simulink model "SABiR_simulator"  (Simulink 8.0)
settings: configuration reference "cset1" (kept outside this file)
values from neighbouring files (symbols this model uses):
  act_Lc_axis1 = act_Phi_axis1 \ acker(act_Phi_axis1', act_H_axis1', poles_Lpr1(1:length(act_Phi_axis1)) )'    [API_setupConstants.m]
  act_Lc_axis2 = act_Phi_axis2 \ acker(act_Phi_axis2', act_H_axis2', poles_Lpr2(1:length(act_Phi_axis2)) )'    [API_setupConstants.m]
  act_Lc_axis3 = act_Phi_axis3 \ acker(act_Phi_axis3', act_H_axis3', poles_Lpr3(1:length(act_Phi_axis3)) )'    [API_setupConstants.m]
  act_Lc_axis4 = act_Phi_axis4 \ acker(act_Phi_axis4', act_H_axis4', poles_Lpr4(1:length(act_Phi_axis4)) )'    [API_setupConstants.m]
  act_Lc_axis5 = act_Phi_axis5 \ acker(act_Phi_axis5', act_H_axis5', poles_Lpr5(1:length(act_Phi_axis5)) )'    [API_setupConstants.m]
  block1MinMax = [-20 0; -240 -180; 340 360]    [API_debugGraphs.m]    (also in API_setupConstants.m)
  block2MinMax = [-12 -7; -220 -200; 345 350]    [API_debugGraphs.m]    (also in API_setupConstants.m)
  est_Gamma_axis1 = [act_Gamma_axis1; 0]    [API_setupConstants.m]
  est_Gamma_axis2 = [act_Gamma_axis2; 0]    [API_setupConstants.m]
  est_Gamma_axis3 = [act_Gamma_axis3; 0]    [API_setupConstants.m]
  est_Gamma_axis4 = [act_Gamma_axis4; 0]    [API_setupConstants.m]
  est_Gamma_axis5 = [act_Gamma_axis5; 0]    [API_setupConstants.m]
  est_H_axis1 = [act_H_axis1, 0]    [API_setupConstants.m]
  est_H_axis2 = [act_H_axis2, 0]    [API_setupConstants.m]
  est_H_axis3 = [act_H_axis3, 0]    [API_setupConstants.m]
  est_H_axis4 = [act_H_axis4, 0]    [API_setupConstants.m]
  est_H_axis5 = [act_H_axis5, 0]    [API_setupConstants.m]
  est_Lc_axis1 = est_Phi_axis1 \ est_Lp_axis1    [API_setupConstants.m]
  est_Lc_axis2 = est_Phi_axis2 \ est_Lp_axis2    [API_setupConstants.m]
  est_Lc_axis3 = est_Phi_axis3 \ est_Lp_axis3    [API_setupConstants.m]
  est_Lc_axis4 = est_Phi_axis4 \ est_Lp_axis4    [API_setupConstants.m]
  est_Lc_axis5 = est_Phi_axis5 \ est_Lp_axis5    [API_setupConstants.m]
  est_Phi_axis1 = [act_Phi_axis1, act_Gamma_axis1; zeros(1,size(act_Phi_axis1,2)), 1]    [API_setupConstants.m]
  est_Phi_axis2 = [act_Phi_axis2, act_Gamma_axis2; zeros(1,size(act_Phi_axis2,2)), 1]    [API_setupConstants.m]
  est_Phi_axis3 = [act_Phi_axis3, act_Gamma_axis3; zeros(1,size(act_Phi_axis3,2)), 1]    [API_setupConstants.m]
  est_Phi_axis4 = [act_Phi_axis4, act_Gamma_axis4; zeros(1,size(act_Phi_axis4,2)), 1]    [API_setupConstants.m]
  est_Phi_axis5 = [act_Phi_axis5, act_Gamma_axis5; zeros(1,size(act_Phi_axis5,2)), 1]    [API_setupConstants.m]
  K_axis1 = acker(act_Phi_axis1, act_Gamma_axis1, poles_Kc1)    [API_setupConstants.m]
  K_axis2 = acker(act_Phi_axis2, act_Gamma_axis2, poles_Kc2)    [API_setupConstants.m]
  K_axis3 = acker(act_Phi_axis3, act_Gamma_axis3, poles_Kc3)    [API_setupConstants.m]
  K_axis4 = acker(act_Phi_axis4, act_Gamma_axis4, poles_Kc4)    [API_setupConstants.m]
  K_axis5 = acker(act_Phi_axis5, act_Gamma_axis5, poles_Kc5)    [API_setupConstants.m]
  Kd_dir = [0;0]    [API_setupConstants.m]
  Kd_pos = [0.0;0.0;0.0]    [API_setupConstants.m]
  Kdir = [12.5; 12.5]    [API_setupConstants.m]
  Kpos = [12.5; 12.5; 12.5]    [API_setupConstants.m]
  Nbar_axis1 = Nu_axis1 + K_axis1 * Nx_axis1    [API_setupConstants.m]
  Nbar_axis2 = Nu_axis2 + K_axis2 * Nx_axis2    [API_setupConstants.m]
  Nbar_axis3 = Nu_axis3 + K_axis3 * Nx_axis3    [API_setupConstants.m]
  Nbar_axis4 = Nu_axis4 + K_axis4 * Nx_axis4    [API_setupConstants.m]
  Nbar_axis5 = Nu_axis5 + K_axis5 * Nx_axis5    [API_setupConstants.m]
  SaturationLowerLimit = -[2;2;2;10;10;0.2]    [API_setupConstants.m]
  SaturationUpperLimit = [2;2;2;10;10;0.2]    [API_setupConstants.m]
  TorqueConstant = [TorqueConstantMotorRE25;     TorqueConstantMotorRE25;     TorqueConstantMotorRE30;     TorqueConstantMotorRE25;     TorqueConstantMotorRE25;     TorqueConstantMotorRE10]./GearRatio    [API_setupConstants.m]
  ts = 0.001    [API_relativeMove.m]    (also in API_setupConstants.m = 0.01; PosRef3D.m; PosRef3D_smooth.m; PosRefConfigSpace.m)
  ts2 = 0.0005    [API_setupConstants.m]
  tsEncoderFailure = TotalTime * encoderFailureTime    [API_simulateRobot.m]
undefined symbols (not defined in the file or in its folder): act_Gamma_axis1, act_Gamma_axis2, act_Gamma_axis3, act_Gamma_axis4, act_Gamma_axis5, act_H_axis1, act_H_axis2, act_H_axis3, act_H_axis4, act_H_axis5, act_Phi_axis1, act_Phi_axis2, act_Phi_axis3, act_Phi_axis4, act_Phi_axis5, den1, den2, den3, den4, den5, DiscIntNeverNeededParam, f_envfilt, J1_r, J2_r, J3_r, J4_r, J5_r, materialParameters1x, materialParameters2x, num1, num2, num3, num4, num5, numEncoderToFail
libraries: simulink x3
(part 1 of 3)
settings Model: Creator=M. Cenk Cavusoglu  LastModifiedBy=zhuofu
settings ConfigSet: SourceLocation=Base Workspace

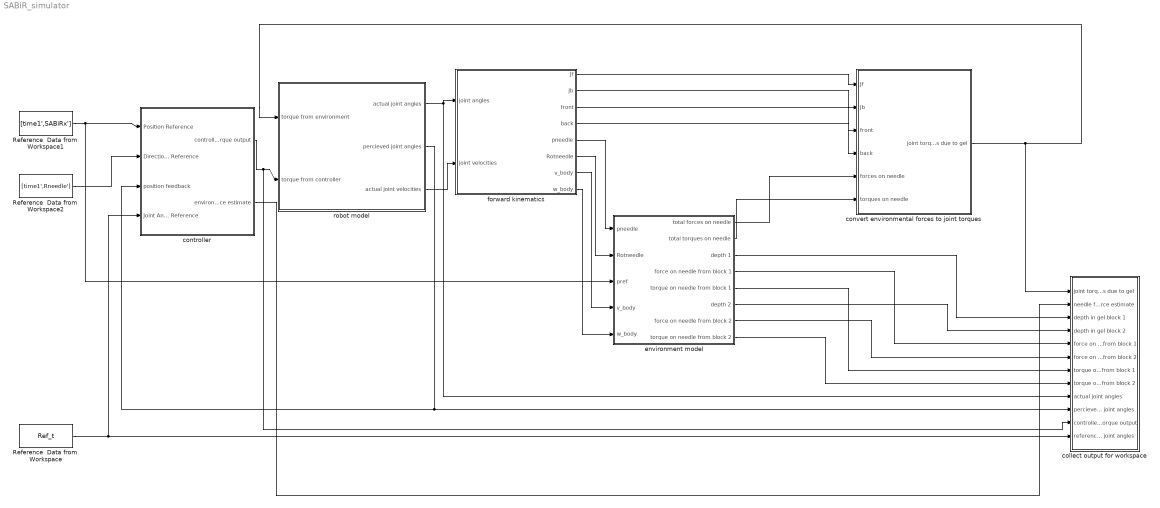
== system SABiR_simulator ==
  Reference  Data from  Workspace : FromWorkspace  VariableName=Ref_t  SampleTime=ts2  OutputAfterFinalValue=Setting to zero
  Reference  Data from  Workspace1 : FromWorkspace  VariableName=[time1',SABiRx']  SampleTime=ts2  OutputAfterFinalValue=Setting to zero
  Reference  Data from  Workspace2 : FromWorkspace  VariableName=[time1',Rneedle']  SampleTime=ts2  OutputAfterFinalValue=Setting to zero
  collect output for workspace : Subsystem
  controller : Subsystem
  convert environmental forces to joint torques : Subsystem
  environment model : Subsystem
  forward kinematics : Subsystem
  robot model : Subsystem
  wires:
  controller/1(controller torque output) -> robot model/2(torque from controller), collect output for workspace/11(controller torque output)
  robot model/2(percieved joint angles) -> collect output for workspace/10(percieved joint angles), controller/3(position feedback)
  convert environmental forces to joint torques/1(joint torques due to gel) -> robot model/1(torque from environment), collect output for workspace/1(joint torques due to gel)
  forward kinematics/1(Jf) -> convert environmental forces to joint torques/1(Jf)
  forward kinematics/2(Jb) -> convert environmental forces to joint torques/2(Jb)
  forward kinematics/5(pneedle) -> environment model/1(pneedle)
  forward kinematics/6(Rotneedle) -> environment model/2(Rotneedle)
  forward kinematics/3(front) -> convert environmental forces to joint torques/3(front)
  forward kinematics/4(back) -> convert environmental forces to joint torques/4(back)
  Reference  Data from  Workspace/1 -> collect output for workspace/12(reference joint angles), controller/4(Joint Angle Reference)
  environment model/1(total forces on needle) -> convert environmental forces to joint torques/5(forces on needle)
  environment model/2(total torques on needle) -> convert environmental forces to joint torques/6(torques on needle)
  environment model/3(depth 1) -> collect output for workspace/3(depth in gel block 1)
  environment model/4(force on needle from block 1) -> collect output for workspace/5(force on needle from block 1)
  environment model/7(force on needle from block 2) -> collect output for workspace/6(force on needle from block 2)
  environment model/5(torque on needle from block 1) -> collect output for workspace/7(torque on needle from block 1)
  environment model/8(torque on needle from block 2) -> collect output for workspace/8(torque on needle from block 2)
  environment model/6(depth 2) -> collect output for workspace/4(depth in gel block 2)
  Reference  Data from  Workspace1/1 -> controller/1(Position Reference), environment model/3(pref)
  Reference  Data from  Workspace2/1 -> controller/2(Direction Reference)
  robot model/1(actual joint angles) -> forward kinematics/1(joint angles), collect output for workspace/9(actual joint angles)
  controller/2(environment force estimate) -> collect output for workspace/2(needle force estimate)
  robot model/3(actual joint velocities) -> forward kinematics/2(joint velocities)
  forward kinematics/7(v_body) -> environment model/4(v_body)
  forward kinematics/8(w_body) -> environment model/5(w_body)

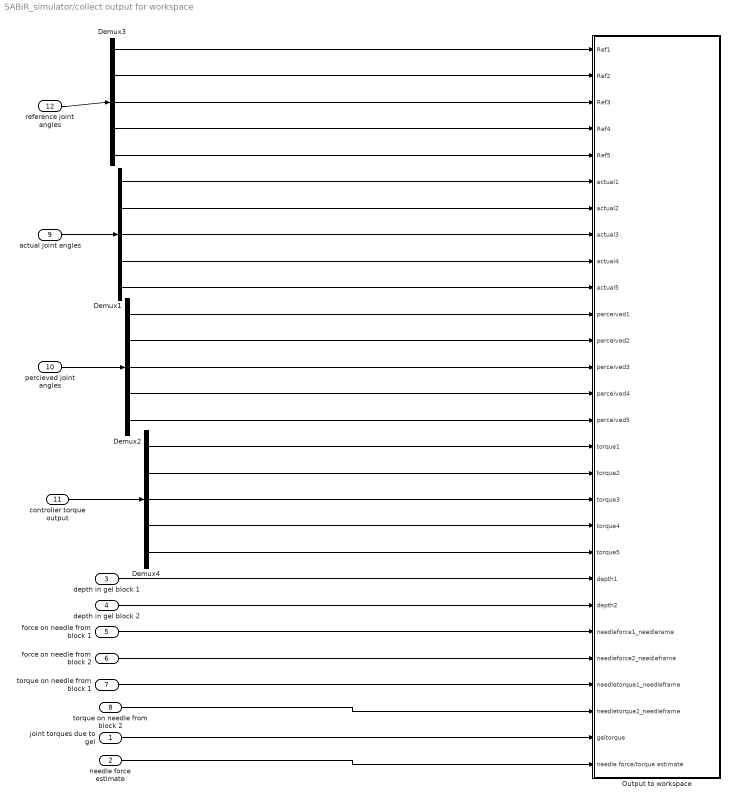
== system SABiR_simulator/collect output for workspace ==
  joint torques due to gel : Inport
  needle force estimate : Inport  Port=2
  depth in gel block 1 : Inport  Port=3
  depth in gel block 2 : Inport  Port=4
  force on needle from block 1 : Inport  Port=5
  force on needle from block 2 : Inport  Port=6
  torque on needle from block 1 : Inport  Port=7
  torque on needle from block 2 : Inport  Port=8
  actual joint angles : Inport  Port=9
  percieved joint angles : Inport  Port=10
  controller torque output : Inport  Port=11
  reference joint angles : Inport  Port=12
  Demux{1..4} (4 alike) : Demux  Outputs=5
  "Output to workspace " : Subsystem
  wires:
  reference joint angles/1 -> Demux3/1
  actual joint angles/1 -> Demux1/1
  percieved joint angles/1 -> Demux2/1
  depth in gel block 1/1 -> "Output to workspace "/21(depth1)
  depth in gel block 2/1 -> "Output to workspace "/22(depth2)
  force on needle from block 1/1 -> "Output to workspace "/23(needleforce1_needlerame)
  force on needle from block 2/1 -> "Output to workspace "/24(needleforce2_needleframe)
  torque on needle from block 1/1 -> "Output to workspace "/25(needletorque1_needleframe)
  torque on needle from block 2/1 -> "Output to workspace "/26(needletorque2_needleframe)
  joint torques due to gel/1 -> "Output to workspace "/27(geltorque)
  Demux3/1 -> "Output to workspace "/1(Ref1)
  Demux3/2 -> "Output to workspace "/2(Ref2)
  Demux3/3 -> "Output to workspace "/3(Ref3)
  Demux3/4 -> "Output to workspace "/4(Ref4)
  Demux3/5 -> "Output to workspace "/5(Ref5)
  Demux1/1 -> "Output to workspace "/6(actual1)
  Demux1/2 -> "Output to workspace "/7(actual2)
  Demux1/3 -> "Output to workspace "/8(actual3)
  Demux1/4 -> "Output to workspace "/9(actual4)
  Demux1/5 -> "Output to workspace "/10(actual5)
  Demux2/1 -> "Output to workspace "/11(perceived1)
  Demux2/2 -> "Output to workspace "/12(perceived2)
  Demux2/3 -> "Output to workspace "/13(perceived3)
  Demux2/4 -> "Output to workspace "/14(perceived4)
  Demux2/5 -> "Output to workspace "/15(perceived5)
  Demux4/1 -> "Output to workspace "/16(torque1)
  Demux4/2 -> "Output to workspace "/17(torque2)
  Demux4/3 -> "Output to workspace "/18(torque3)
  Demux4/4 -> "Output to workspace "/19(torque4)
  Demux4/5 -> "Output to workspace "/20(torque5)
  controller torque output/1 -> Demux4/1
  needle force estimate/1 -> "Output to workspace "/28(needle force/torque estimate)

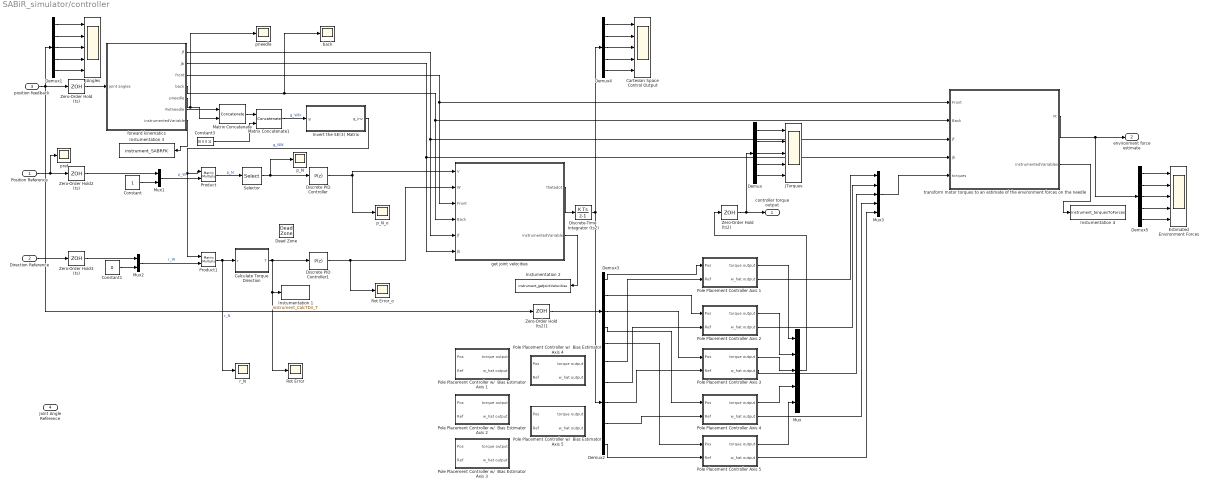
== system SABiR_simulator/controller ==
  Position Reference : Inport
  Direction Reference : Inport  Port=2
  position feedback : Inport  Port=3
  Joint Angle Reference : Inport  Port=4
  Calculate Torque Direction : MATLAB Function  TreatAsAtomicUnit=on
  Cartesian Space Control Output : Scope  NumInputPorts=5
      settings: TimeRange=5  YMin=-1~-1~-7500~-1500~-200  YMax=1~1~10000~250~1000  SaveName=ScopeData15  MaxDataPoints=50000
  Constant : Constant
  Constant1 : Constant  Value=0
  Constant3 : Constant  Value=[0 0 0 1]  VectorParams1D=off
  Dead Zone : DeadZone  LowerValue=-[0;0;0.05]  UpperValue=[0;0;0.05]  SaturateOnIntegerOverflow=on
  Demux{,1..5} (6 alike) : Demux  Outputs=5
  Discrete PID Controller : simulink/Continuous/PID Controller  Controller=P  TimeDomain=Discrete-time  SampleTime=ts  IntegratorMethod=Forward Euler  FilterMethod=Forward Euler  Form=Ideal  P=Kpos  I=0  D=Kd_pos  N=100  InitialConditionSource=internal  InitialConditionForIntegrator=0  InitialConditionForFilter=0  ExternalReset=none  LimitOutput=off  UpperSaturationLimit=inf  LowerSaturationLimit=-inf  LinearizeAsGain=off  AntiWindupMode=none  Kb=1  TrackingMode=off  Kt=1  PParamMin=[]  PParamMax=[]  IParamMin=[]  IParamMax=[]  DParamMin=[]  DParamMax=[]  NParamMin=[]  NParamMax=[]  KbParamMin=[]  KbParamMax=[]  KtParamMin=[]  KtParamMax=[]  POutMin=[]  POutMax=[]  IOutMin=[]  IOutMax=[]  DOutMin=[]  DOutMax=[]  NOutMin=[]  NOutMax=[]  KbOutMin=[]  KbOutMax=[]  KtOutMin=[]  KtOutMax=[]  IntegratorOutMin=[]  IntegratorOutMax=[]  FilterOutMin=[]  FilterOutMax=[]  SumOutMin=[]  SumOutMax=[]  SumI1OutMin=[]  SumI1OutMax=[]  SumI2OutMin=[]  SumI2OutMax=[]  SumI3OutMin=[]  SumI3OutMax=[]  SumDOutMin=[]  SumDOutMax=[]  SaturationOutMin=[]  SaturationOutMax=[]  IntegratorContinuousStateAttributes=''  IntegratorStateMustResolveToSignalObject=off  IntegratorRTWStateStorageClass=Auto  FilterContinuousStateAttributes=''  FilterStateMustResolveToSignalObject=off  FilterRTWStateStorageClass=Auto
  Discrete PID Controller1 : simulink/Continuous/PID Controller  Controller=P  TimeDomain=Discrete-time  SampleTime=ts  IntegratorMethod=Forward Euler  FilterMethod=Forward Euler  Form=Ideal  P=Kdir  I=0  D=Kd_dir  N=100  InitialConditionSource=internal  InitialConditionForIntegrator=0  InitialConditionForFilter=0  ExternalReset=none  LimitOutput=off  UpperSaturationLimit=inf  LowerSaturationLimit=-inf  LinearizeAsGain=off  AntiWindupMode=none  Kb=1  TrackingMode=off  Kt=1  PParamMin=[]  PParamMax=[]  IParamMin=[]  IParamMax=[]  DParamMin=[]  DParamMax=[]  NParamMin=[]  NParamMax=[]  KbParamMin=[]  KbParamMax=[]  KtParamMin=[]  KtParamMax=[]  POutMin=[]  POutMax=[]  IOutMin=[]  IOutMax=[]  DOutMin=[]  DOutMax=[]  NOutMin=[]  NOutMax=[]  KbOutMin=[]  KbOutMax=[]  KtOutMin=[]  KtOutMax=[]  IntegratorOutMin=[]  IntegratorOutMax=[]  FilterOutMin=[]  FilterOutMax=[]  SumOutMin=[]  SumOutMax=[]  SumI1OutMin=[]  SumI1OutMax=[]  SumI2OutMin=[]  SumI2OutMax=[]  SumI3OutMin=[]  SumI3OutMax=[]  SumDOutMin=[]  SumDOutMax=[]  SaturationOutMin=[]  SaturationOutMax=[]  IntegratorContinuousStateAttributes=''  IntegratorStateMustResolveToSignalObject=off  IntegratorRTWStateStorageClass=Auto  FilterContinuousStateAttributes=''  FilterStateMustResolveToSignalObject=off  FilterRTWStateStorageClass=Auto
  Discrete-Time Integrator (ts2) : DiscreteIntegrator  SampleTime=ts2  ICPrevOutput=DiscIntNeverNeededParam  ICPrevScaledInput=DiscIntNeverNeededParam
  Estimated Environment Forces : Scope  NumInputPorts=5
      settings: TimeRange=17.98  YMin=-5e-005~-1.75e-005~-0.0013~-0.006~-0.02  YMax=6e-005~1.25e-005~0.0001~0.004~0.0175  SaveName=ScopeData31  MaxDataPoints=50000
  Instumentation 1 : ToWorkspace  VariableName=instrument_CalcTDir_T  SampleTime=-1  SaveFormat=Structure
  Instumentation 2 : ToWorkspace  VariableName=instrument_getJointVelocities  SampleTime=-1  SaveFormat=Structure
  Instumentation 3 : ToWorkspace  VariableName=instrument_SABRFK  SampleTime=-1  SaveFormat=Structure
  Instumentation 4 : ToWorkspace  VariableName=instrument_torquesToForces  SampleTime=-1  SaveFormat=Structure
  Invert the SE(3) Matrix : MATLAB Function  TreatAsAtomicUnit=on
  JAngles : Scope  NumInputPorts=5
      settings: TimeRange=0.05  YMin=-1~-1~-3.511231084753035e-007~-1~-1  YMax=1~1~2.015504774369832e-007~1~1  SaveName=ScopeData6  MaxDataPoints=50000
  JTorques : Scope  NumInputPorts=5
      settings: TimeRange=18  YMin=-0.00025~-0.0003~-0.0003~-0.0007~-0.00075  YMax=0.0002~0.0003~0.00015~0.0004~0.001  SaveName=ScopeData3  MaxDataPoints=50000
  Matrix Concatenate : Concatenate  Mode=Multidimensional array  ConcatenateDimension=2
  Matrix Concatenate1 : Concatenate  Mode=Multidimensional array
  Mux : Mux  Inputs=5
  Mux1 : Mux  Inputs=[3 1]
  Mux2 : Mux  Inputs=[3 1]
  Mux3 : Mux  Inputs=5
  Pole Placement Controller Axis 1 : Subsystem
  Pole Placement Controller Axis 2 : Subsystem
  Pole Placement Controller Axis 3 : Subsystem
  Pole Placement Controller Axis 4 : Subsystem
  Pole Placement Controller Axis 5 : Subsystem
  Pole Placement Controller w/  Bias Estimator Axis 1 : Subsystem
  Pole Placement Controller w/  Bias Estimator Axis 2 : Subsystem
  Pole Placement Controller w/  Bias Estimator Axis 3 : Subsystem
  Pole Placement Controller w/  Bias Estimator Axis 4 : Subsystem
  Pole Placement Controller w/  Bias Estimator Axis 5 : Subsystem
  Product : Product  Multiplication=Matrix(*)  RndMeth=Zero
  Product1 : Product  Multiplication=Matrix(*)  RndMeth=Zero
  Rot Error : Scope
      settings: TimeRange=12  YMin=-0.15  YMax=0.55  SaveName=ScopeData2  MaxDataPoints=50000
  Rot Error_o : Scope
      settings: TimeRange=5  YMin=-150  YMax=100  SaveName=ScopeData17  MaxDataPoints=50000
  Selector : Selector  InputPortWidth=4  IndexOptions=Index vector (dialog)  Indices=[1 2 3]  OutputSizes=1
  Zero-Order Hold (ts) : ZeroOrderHold  SampleTime=ts
  Zero-Order Hold (ts2) : ZeroOrderHold  SampleTime=ts2
  Zero-Order Hold (ts2)1 : ZeroOrderHold  SampleTime=ts2
  Zero-Order Hold2 (ts) : ZeroOrderHold  SampleTime=ts
  Zero-Order Hold3 (ts) : ZeroOrderHold  SampleTime=ts
  back : Scope
      settings: TimeRange=5  YMin=-150  YMax=100  SaveName=ScopeData5  MaxDataPoints=50000
  forward kinematics : Subsystem
  get joint velocities : MATLAB Function  TreatAsAtomicUnit=on
  p_N : Scope
      settings: TimeRange=17.98  YMin=-0.55  YMax=0.55  MaxDataPoints=50000
  p_N_o : Scope
      settings: TimeRange=5  YMin=-150  YMax=100  SaveName=ScopeData16  MaxDataPoints=50000
  pneedle : Scope
      settings: TimeRange=17.98  YMin=-225  YMax=350  SaveName=ScopeData4  MaxDataPoints=50000
  pref : Scope
      settings: TimeRange=17.98  YMin=-225  YMax=350  SaveName=ScopeData21  MaxDataPoints=50000
  r_N : Scope
      settings: TimeRange=5  YMin=-150  YMax=100  MaxDataPoints=50000
  transform motor torques to an estimate of the environment forces on the needle : MATLAB Function  TreatAsAtomicUnit=on
  controller torque output : Outport
  environment force estimate : Outport  Port=2
  wires:
  Position Reference/1 -> Zero-Order Hold2 (ts)/1, pref/1
  position feedback/1 -> Zero-Order Hold (ts)/1, Demux1/1, Zero-Order Hold (ts2)1/1
  Direction Reference/1 -> Zero-Order Hold3 (ts)/1
  Matrix Concatenate1/1 -> Invert the SE(3) Matrix/1(g)  "g_WN"
  Zero-Order Hold2 (ts)/1 -> Mux1/1
  Constant/1 -> Mux1/2
  Invert the SE(3) Matrix/1(g_inv) -> Product/1, Product1/1  "g_NW"
  Mux1/1 -> Product/2  "p_W"
  Product/1 -> Selector/1  "p_N"
  Selector/1 -> p_N/1, Discrete PID Controller/1
  Constant1/1 -> Mux2/2
  Zero-Order Hold3 (ts)/1 -> Mux2/1
  Mux2/1 -> Product1/2  "r_W"
  Product1/1 -> Calculate Torque Direction/1(r), r_N/1  "r_N"
  Calculate Torque Direction/1(T) -> Discrete PID Controller1/1, Rot Error/1, Instumentation 1/1
  Discrete PID Controller1/1 -> Rot Error_o/1, get joint velocities/2(W)
  forward kinematics/3(front) -> get joint velocities/3(Front), transform motor torques to an estimate of the environment forces on the needle/1(Front)
  forward kinematics/4(back) -> back/1, get joint velocities/4(Back), transform motor torques to an estimate of the environment forces on the needle/2(Back)
  forward kinematics/1(Jf) -> get joint velocities/5(Jf), transform motor torques to an estimate of the environment forces on the needle/3(Jf)
  forward kinematics/2(Jb) -> get joint velocities/6(Jb), transform motor torques to an estimate of the environment forces on the needle/4(Jb)
  forward kinematics/6(Rotneedle) -> Matrix Concatenate/1
  forward kinematics/5(pneedle) -> pneedle/1, Matrix Concatenate/2
  Matrix Concatenate/1 -> Matrix Concatenate1/1
  Constant3/1 -> Matrix Concatenate1/2
  Demux/5 -> JTorques/5
  Demux/4 -> JTorques/4
  Demux/3 -> JTorques/3
  Demux/2 -> JTorques/2
  Demux/1 -> JTorques/1
  Demux1/5 -> JAngles/5
  Demux1/4 -> JAngles/4
  Demux1/3 -> JAngles/3
  Demux1/2 -> JAngles/2
  Demux1/1 -> JAngles/1
  Discrete PID Controller/1 -> p_N_o/1, get joint velocities/1(V)
  Pole Placement Controller Axis 4/1(torque output) -> Mux/4
  Pole Placement Controller Axis 5/1(torque output) -> Mux/5
  Pole Placement Controller Axis 3/1(torque output) -> Mux/3
  Pole Placement Controller Axis 2/1(torque output) -> Mux/2
  Pole Placement Controller Axis 1/1(torque output) -> Mux/1
  Demux2/5 -> Pole Placement Controller Axis 5/2(Ref)
  Demux2/4 -> Pole Placement Controller Axis 4/2(Ref)
  Demux2/3 -> Pole Placement Controller Axis 3/2(Ref)
  Demux2/2 -> Pole Placement Controller Axis 2/2(Ref)
  Demux2/1 -> Pole Placement Controller Axis 1/2(Ref)
  Demux3/1 -> Pole Placement Controller Axis 1/1(Pos)
  Demux3/2 -> Pole Placement Controller Axis 2/1(Pos)
  Demux3/3 -> Pole Placement Controller Axis 3/1(Pos)
  Demux3/4 -> Pole Placement Controller Axis 4/1(Pos)
  Demux3/5 -> Pole Placement Controller Axis 5/1(Pos)
  Demux4/5 -> Cartesian Space Control Output/5
  Demux4/4 -> Cartesian Space Control Output/4
  Demux4/3 -> Cartesian Space Control Output/3
  Demux4/2 -> Cartesian Space Control Output/2
  Demux4/1 -> Cartesian Space Control Output/1
  Zero-Order Hold (ts2)/1 -> controller torque output/1, Demux/1
  Mux/1 -> Zero-Order Hold (ts2)/1
  get joint velocities/1(thetadot) -> Discrete-Time Integrator (ts2)/1
  Discrete-Time Integrator (ts2)/1 -> Demux4/1, Demux2/1
  Zero-Order Hold (ts)/1 -> forward kinematics/1(joint angles)
  Zero-Order Hold (ts2)1/1 -> Demux3/1
  transform motor torques to an estimate of the environment forces on the needle/1(Ft) -> environment force estimate/1, Demux5/1
  Mux3/1 -> transform motor torques to an estimate of the environment forces on the needle/5(torques)
  Pole Placement Controller Axis 5/2(w_hat output) -> Mux3/5
  Pole Placement Controller Axis 4/2(w_hat output) -> Mux3/4
  Pole Placement Controller Axis 2/2(w_hat output) -> Mux3/2
  Pole Placement Controller Axis 1/2(w_hat output) -> Mux3/1
  Pole Placement Controller Axis 3/2(w_hat output) -> Mux3/3
  Demux5/5 -> Estimated Environment Forces/5
  Demux5/4 -> Estimated Environment Forces/4
  Demux5/3 -> Estimated Environment Forces/3
  Demux5/2 -> Estimated Environment Forces/2
  Demux5/1 -> Estimated Environment Forces/1
  get joint velocities/2(instrumentedVariable) -> Instumentation 2/1
  transform motor torques to an estimate of the environment forces on the needle/2(instrumentedVariables) -> Instumentation 4/1
  forward kinematics/7(instrumentedVariable) -> Instumentation 3/1

== system SABiR_simulator/convert environmental forces to joint torques ==
  Jf : Inport
  Jb : Inport  Port=2
  front : Inport  Port=3
  back : Inport  Port=4
  forces on needle : Inport  Port=5
  torques on needle : Inport  Port=6
  Demux1 : Demux  Outputs=3
  Demux2 : Demux  Outputs=3
  Env Forces on Needle : Scope  NumInputPorts=3
      settings: TimeRange=17.98  YMin=-7.5e-007~-7e-007~-0.0013  YMax=2e-006~3e-007~0.0001  SaveName=ScopeData32  MaxDataPoints=50000
  Env Torques on Needle : Scope  NumInputPorts=3
      settings: TimeRange=17.98  YMin=-2.75e-008~-1.2e-007~-1e-008  YMax=1e-008~1e-008~5e-009  SaveName=ScopeData33  MaxDataPoints=50000
  Motor Torques Due to Environment Forces : Scope
      settings: TimeRange=17.98  YMin=-1  YMax=1  SaveName=ScopeData22  MaxDataPoints=50000
  get joint torques : MATLAB Function  TreatAsAtomicUnit=on
  joint torques due to gel : Outport
  wires:
  forces on needle/1 -> get joint torques/1(F), Demux2/1
  torques on needle/1 -> get joint torques/2(T), Demux1/1
  front/1 -> get joint torques/3(Front)
  back/1 -> get joint torques/4(Back)
  Jf/1 -> get joint torques/5(Jf)
  Jb/1 -> get joint torques/6(Jb)
  get joint torques/1(torques) -> joint torques due to gel/1, Motor Torques Due to Environment Forces/1
  Demux1/3 -> Env Torques on Needle/3
  Demux1/2 -> Env Torques on Needle/2
  Demux1/1 -> Env Torques on Needle/1
  Demux2/3 -> Env Forces on Needle/3
  Demux2/2 -> Env Forces on Needle/2
  Demux2/1 -> Env Forces on Needle/1

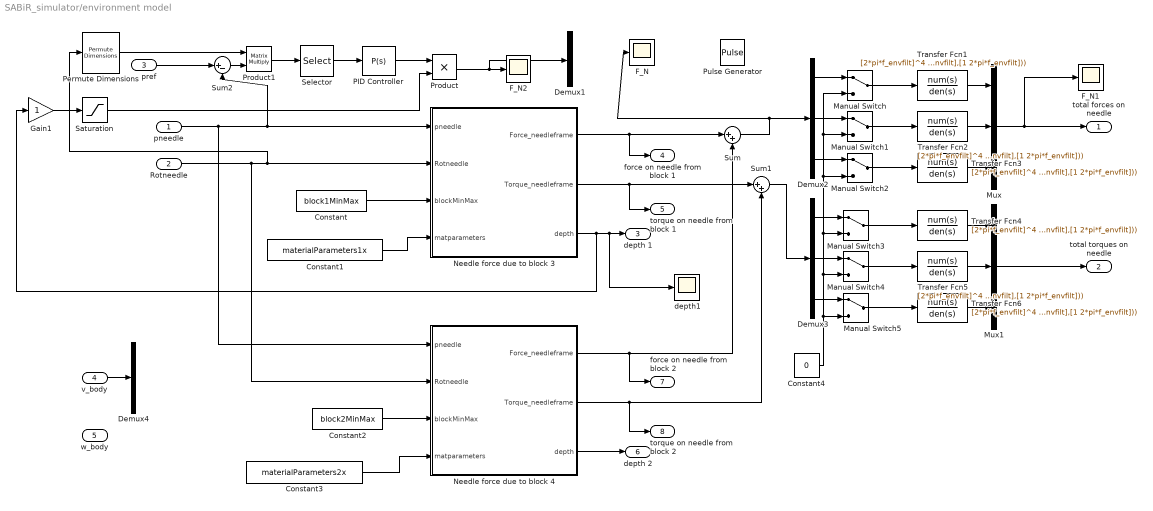
== system SABiR_simulator/environment model ==
  pneedle : Inport
  Rotneedle : Inport  Port=2
  pref : Inport  Port=3
  v_body : Inport  Port=4
  w_body : Inport  Port=5
  Constant : Constant  Value=block1MinMax  VectorParams1D=off
  Constant1 : Constant  Value=materialParameters1x  VectorParams1D=off
  Constant2 : Constant  Value=block2MinMax  VectorParams1D=off
  Constant3 : Constant  Value=materialParameters2x  VectorParams1D=off
  Constant4 : Constant  Value=0
  Demux1 : Demux  Outputs=2
  Demux2 : Demux  Outputs=3
  Demux3 : Demux  Outputs=3
  Demux4 : Demux  Outputs=3
  F_N : Scope
      settings: TimeRange=5  YMin=-0.175  YMax=0.1  SaveName=ScopeData23  MaxDataPoints=50000
  F_N1 : Scope
      settings: TimeRange=17.98  YMin=-1  YMax=1  SaveName=ScopeData24  MaxDataPoints=50000
  F_N2 : Scope
      settings: TimeRange=5  YMin=-1.75e-005  YMax=1.75e-005  SaveName=ScopeData26  MaxDataPoints=50000
  Gain1 : Gain
  Manual Switch{,1..5} (6 alike) : ManualSwitch
  Mux : Mux  Inputs=3
  Mux1 : Mux  Inputs=3
  Needle force due to block 3 : Subsystem
  Needle force due to block 4 : Subsystem
  PID Controller : simulink/Continuous/PID Controller  Controller=P  TimeDomain=Continuous-time  SampleTime=1  IntegratorMethod=Forward Euler  FilterMethod=Forward Euler  Form=Ideal  P=0.0087/25  I=0  D=0  N=100  InitialConditionSource=internal  InitialConditionForIntegrator=0  InitialConditionForFilter=0  ExternalReset=none  LimitOutput=off  UpperSaturationLimit=inf  LowerSaturationLimit=-inf  LinearizeAsGain=off  AntiWindupMode=none  Kb=1  TrackingMode=off  Kt=1  PParamMin=[]  PParamMax=[]  IParamMin=[]  IParamMax=[]  DParamMin=[]  DParamMax=[]  NParamMin=[]  NParamMax=[]  KbParamMin=[]  KbParamMax=[]  KtParamMin=[]  KtParamMax=[]  POutMin=[]  POutMax=[]  IOutMin=[]  IOutMax=[]  DOutMin=[]  DOutMax=[]  NOutMin=[]  NOutMax=[]  KbOutMin=[]  KbOutMax=[]  KtOutMin=[]  KtOutMax=[]  IntegratorOutMin=[]  IntegratorOutMax=[]  FilterOutMin=[]  FilterOutMax=[]  SumOutMin=[]  SumOutMax=[]  SumI1OutMin=[]  SumI1OutMax=[]  SumI2OutMin=[]  SumI2OutMax=[]  SumI3OutMin=[]  SumI3OutMax=[]  SumDOutMin=[]  SumDOutMax=[]  SaturationOutMin=[]  SaturationOutMax=[]  IntegratorContinuousStateAttributes=''  IntegratorStateMustResolveToSignalObject=off  IntegratorRTWStateStorageClass=Auto  FilterContinuousStateAttributes=''  FilterStateMustResolveToSignalObject=off  FilterRTWStateStorageClass=Auto
  Permute Dimensions : PermuteDimensions
  Product : Product  RndMeth=Zero
  Product1 : Product  Multiplication=Matrix(*)  RndMeth=Zero
  Pulse Generator : DiscretePulseGenerator  PulseType=Time based  Amplitude=1e-5  Period=1  PulseWidth=5
  Saturation : Saturate  UpperLimit=20  LowerLimit=0
  Selector : Selector  InputPortWidth=3  IndexOptions=Index vector (dialog)  Indices=[1 2]  OutputSizes=1
  Sum : Sum  Inputs=|++
  Sum1 : Sum  Inputs=|++
  Sum2 : Sum  Inputs=|+-
  Transfer Fcn{1..6} (6 alike) : TransferFcn  Numerator=[2*pi*f_envfilt]^4  Denominator=conv(conv([1 2*pi*f_envfilt],[1 2*pi*f_envfilt]),conv([1 2*pi*f_envfilt],[1 2*pi*f_envfilt]))
  depth1 : Scope
      settings: TimeRange=5  YMin=-0.175  YMax=0.1  SaveName=ScopeData25  MaxDataPoints=50000
  total forces on needle : Outport
  total torques on needle : Outport  Port=2
  depth 1 : Outport  Port=3
  force on needle from block 1 : Outport  Port=4
  torque on needle from block 1 : Outport  Port=5
  depth 2 : Outport  Port=6
  force on needle from block 2 : Outport  Port=7
  torque on needle from block 2 : Outport  Port=8
  wires:
  pneedle/1 -> Sum2/2, Needle force due to block 3/1(pneedle), Needle force due to block 4/1(pneedle)
  Rotneedle/1 -> Permute Dimensions/1, Needle force due to block 3/2(Rotneedle), Needle force due to block 4/2(Rotneedle)
  Needle force due to block 3/3(depth) -> Gain1/1, depth 1/1, depth1/1
  Needle force due to block 3/1(Force_needleframe) -> Sum/1, force on needle from block 1/1
  Needle force due to block 3/2(Torque_needleframe) -> Sum1/1, torque on needle from block 1/1
  Needle force due to block 4/3(depth) -> depth 2/1
  Needle force due to block 4/1(Force_needleframe) -> force on needle from block 2/1, Sum/2
  Needle force due to block 4/2(Torque_needleframe) -> torque on needle from block 2/1, Sum1/2
  Constant/1 -> Needle force due to block 3/3(blockMinMax)
  Constant2/1 -> Needle force due to block 4/3(blockMinMax)
  Constant3/1 -> Needle force due to block 4/4(matparameters)
  Mux/1 -> F_N1/1, total forces on needle/1
  Mux1/1 -> total torques on needle/1
  Manual Switch/1 -> Transfer Fcn1/1
  Manual Switch1/1 -> Transfer Fcn2/1
  Manual Switch3/1 -> Transfer Fcn4/1
  Manual Switch4/1 -> Transfer Fcn5/1
  Manual Switch5/1 -> Transfer Fcn6/1
  Sum1/1 -> Demux3/1
  Sum/1 -> F_N/1, Demux2/1
  Demux2/3 -> Manual Switch2/1
  Demux3/1 -> Manual Switch3/1
  Demux3/2 -> Manual Switch4/1
  Demux3/3 -> Manual Switch5/1
  Constant4/1 -> Manual Switch5/2, Manual Switch4/2, Manual Switch3/2, Manual Switch2/2, Manual Switch1/2, Manual Switch/2
  Saturation/1 -> Product/2
  PID Controller/1 -> Product/1
  Product/1 -> F_N2/1, Demux1/1
  Gain1/1 -> Saturation/1
  Selector/1 -> PID Controller/1
  Product1/1 -> Selector/1
  Sum2/1 -> Product1/2
  Permute Dimensions/1 -> Product1/1
  pref/1 -> Sum2/1
  Constant1/1 -> Needle force due to block 3/4(matparameters)
  Demux2/2 -> Manual Switch1/1
  Demux2/1 -> Manual Switch/1
  Manual Switch2/1 -> Transfer Fcn3/1
  v_body/1 -> Demux4/1
  Transfer Fcn1/1 -> Mux/1
  Transfer Fcn2/1 -> Mux/2
  Transfer Fcn3/1 -> Mux/3
  Transfer Fcn4/1 -> Mux1/1
  Transfer Fcn5/1 -> Mux1/2
  Transfer Fcn6/1 -> Mux1/3

== system SABiR_simulator/forward kinematics ==
  joint angles : Inport
  joint velocities : Inport  Port=2
  Bus Selector : BusSelector  OutputSignals=signal1,signal2,signal3,signal4,signal5
  Demux4 : Demux  Outputs=6
  Needle Body Velociy : Scope  NumInputPorts=5
      settings: TimeRange=17.98  YMin=-45~-10~-125~-0.07~-0.3  YMax=40~10~100~0.06~0.3  SaveName=ScopeData28  MaxDataPoints=50000
  forward kinematics1 : MATLAB Function  TreatAsAtomicUnit=on
  get joint velocities : MATLAB Function  TreatAsAtomicUnit=on
  Jf : Outport
  Jb : Outport  Port=2
  front : Outport  Port=3
  back : Outport  Port=4
  pneedle : Outport  Port=5
  Rotneedle : Outport  Port=6
  v_body : Outport  Port=7
  w_body : Outport  Port=8
  wires:
  forward kinematics1/1(NeedleTip) -> pneedle/1
  forward kinematics1/3(Front) -> front/1, get joint velocities/2(Front)
  forward kinematics1/4(Back) -> back/1, get joint velocities/3(Back)
  forward kinematics1/5(Jf) -> Jf/1, get joint velocities/4(Jf)
  forward kinematics1/6(Jb) -> Jb/1, get joint velocities/5(Jb)
  forward kinematics1/2(NeedleRot) -> Rotneedle/1
  joint angles/1 -> Bus Selector/1
  Bus Selector/1 -> forward kinematics1/1(t1)  "<signal1>"
  Bus Selector/2 -> forward kinematics1/2(t2)  "<signal2>"
  Bus Selector/3 -> forward kinematics1/3(t3)  "<signal3>"
  Bus Selector/4 -> forward kinematics1/4(t4)  "<signal4>"
  Bus Selector/5 -> forward kinematics1/5(t5)  "<signal5>"
  joint velocities/1 -> get joint velocities/1(thetadot)
  get joint velocities/2(wb) -> w_body/1
  get joint velocities/1(vb) -> v_body/1
  Demux4/5 -> Needle Body Velociy/5
  Demux4/4 -> Needle Body Velociy/4
  Demux4/3 -> Needle Body Velociy/3
  Demux4/2 -> Needle Body Velociy/2
  Demux4/1 -> Needle Body Velociy/1
  get joint velocities/3(bodyVel) -> Demux4/1

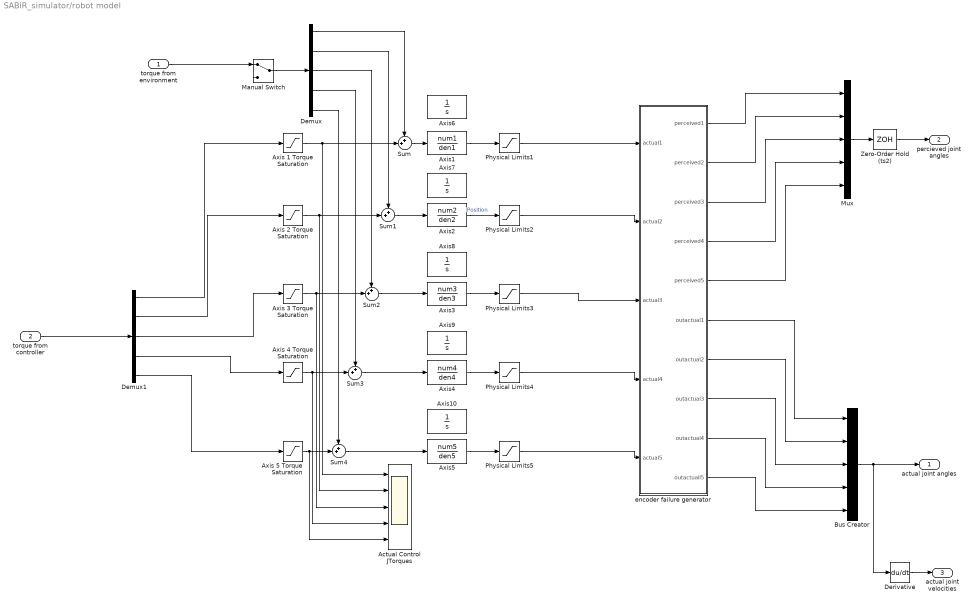
== system SABiR_simulator/robot model ==
  torque from environment : Inport
  torque from controller : Inport  Port=2
  Actual Control JTorques : Scope  NumInputPorts=5
      settings: TimeRange=5  YMin=-0.0001~-2e-005~-1e-005~-0.0003~-7.5e-005  YMax=0.000225~0.00014~0.00011~0.0008~0.000275  SaveName=ScopeData20  MaxDataPoints=50000
  Axis 1 Torque Saturation : Saturate  UpperLimit=SaturationUpperLimit(1)./(1./TorqueConstant(1))  LowerLimit=SaturationLowerLimit(1)./(1./TorqueConstant(1))
  Axis 2 Torque Saturation : Saturate  UpperLimit=SaturationUpperLimit(2)./(1./TorqueConstant(2))  LowerLimit=SaturationLowerLimit(2)./(1./TorqueConstant(2))
  Axis 3 Torque Saturation : Saturate  UpperLimit=SaturationUpperLimit(3)./(1./TorqueConstant(3))  LowerLimit=SaturationLowerLimit(3)./(1./TorqueConstant(3))
  Axis 4 Torque Saturation : Saturate  UpperLimit=SaturationUpperLimit(4)./(1./TorqueConstant(4))  LowerLimit=SaturationLowerLimit(4)./(1./TorqueConstant(4))
  Axis 5 Torque Saturation : Saturate  UpperLimit=SaturationUpperLimit(5)./(1./TorqueConstant(5))  LowerLimit=SaturationLowerLimit(5)./(1./TorqueConstant(5))
  Axis1 : TransferFcn  Numerator=num1  Denominator=den1
  Axis10 : TransferFcn  Denominator=[1 0]
  Axis2 : TransferFcn  Numerator=num2  Denominator=den2
  Axis3 : TransferFcn  Numerator=num3  Denominator=den3  ContinuousStateAttributes='tf3'
  Axis4 : TransferFcn  Numerator=num4  Denominator=den4
  Axis5 : TransferFcn  Numerator=num5  Denominator=den5
  Axis{6..9} (4 alike) : TransferFcn  Numerator=1  Denominator=[1 0]
  Bus Creator : BusCreator  Inputs=5
  Demux : Demux  Outputs=5
  Demux1 : Demux  Outputs=5
  Derivative : Derivative
  Manual Switch : ManualSwitch
  Mux : Mux  Inputs=5
  Physical Limits1 : Saturate  UpperLimit=0.7854  LowerLimit=-0.5060
  Physical Limits2 : Saturate  UpperLimit=0.4841  LowerLimit=-0.7854
  Physical Limits3 : Saturate  UpperLimit=0.2961*100  LowerLimit=-0.2618*100
  Physical Limits4 : Saturate  UpperLimit=0.7854  LowerLimit=-0.4531
  Physical Limits5 : Saturate  UpperLimit=0.4396  LowerLimit=-0.7854
  Sum{,1..4} (5 alike) : Sum  Inputs=++|
  Zero-Order Hold (ts2) : ZeroOrderHold  SampleTime=ts2
  encoder failure generator : Subsystem
  actual joint angles : Outport
  percieved joint angles : Outport  Port=2
  actual joint velocities : Outport  Port=3
  wires:
  Axis 3 Torque Saturation/1 -> Sum2/2, Actual Control JTorques/3
  Physical Limits1/1 -> encoder failure generator/1(actual1)
  Physical Limits2/1 -> encoder failure generator/2(actual2)
  Physical Limits4/1 -> encoder failure generator/4(actual4)
  Physical Limits5/1 -> encoder failure generator/5(actual5)
  torque from controller/1 -> Demux1/1
  Demux1/3 -> Axis 3 Torque Saturation/1
  Demux/1 -> Sum/1
  Demux/2 -> Sum1/1
  Demux/3 -> Sum2/1
  Demux/4 -> Sum3/1
  Demux/5 -> Sum4/1
  Axis 1 Torque Saturation/1 -> Sum/2, Actual Control JTorques/1
  Axis 2 Torque Saturation/1 -> Sum1/2, Actual Control JTorques/2
  Axis 4 Torque Saturation/1 -> Sum3/2, Actual Control JTorques/4
  Axis 5 Torque Saturation/1 -> Sum4/2, Actual Control JTorques/5
  Mux/1 -> Zero-Order Hold (ts2)/1
  encoder failure generator/1(perceived1) -> Mux/1
  encoder failure generator/2(perceived2) -> Mux/2
  encoder failure generator/3(perceived3) -> Mux/3
  encoder failure generator/4(perceived4) -> Mux/4
  encoder failure generator/5(perceived5) -> Mux/5
  Physical Limits3/1 -> encoder failure generator/3(actual3)
  Zero-Order Hold (ts2)/1 -> percieved joint angles/1
  torque from environment/1 -> Manual Switch/1
  Manual Switch/1 -> Demux/1
  Demux1/5 -> Axis 5 Torque Saturation/1
  Demux1/4 -> Axis 4 Torque Saturation/1
  Demux1/2 -> Axis 2 Torque Saturation/1
  Demux1/1 -> Axis 1 Torque Saturation/1
  Sum/1 -> Axis1/1
  Axis1/1 -> Physical Limits1/1
  Sum1/1 -> Axis2/1
  Axis2/1 -> Physical Limits2/1  "Position"
  Sum2/1 -> Axis3/1
  Axis3/1 -> Physical Limits3/1
  Sum3/1 -> Axis4/1
  Axis4/1 -> Physical Limits4/1
  Sum4/1 -> Axis5/1
  Axis5/1 -> Physical Limits5/1
  encoder failure generator/6(outactual1) -> Bus Creator/1
  encoder failure generator/7(outactual2) -> Bus Creator/2
  encoder failure generator/8(outactual3) -> Bus Creator/3
  encoder failure generator/9(outactual4) -> Bus Creator/4
  encoder failure generator/10(outactuall5) -> Bus Creator/5
  Bus Creator/1 -> actual joint angles/1, Derivative/1
  Derivative/1 -> actual joint velocities/1

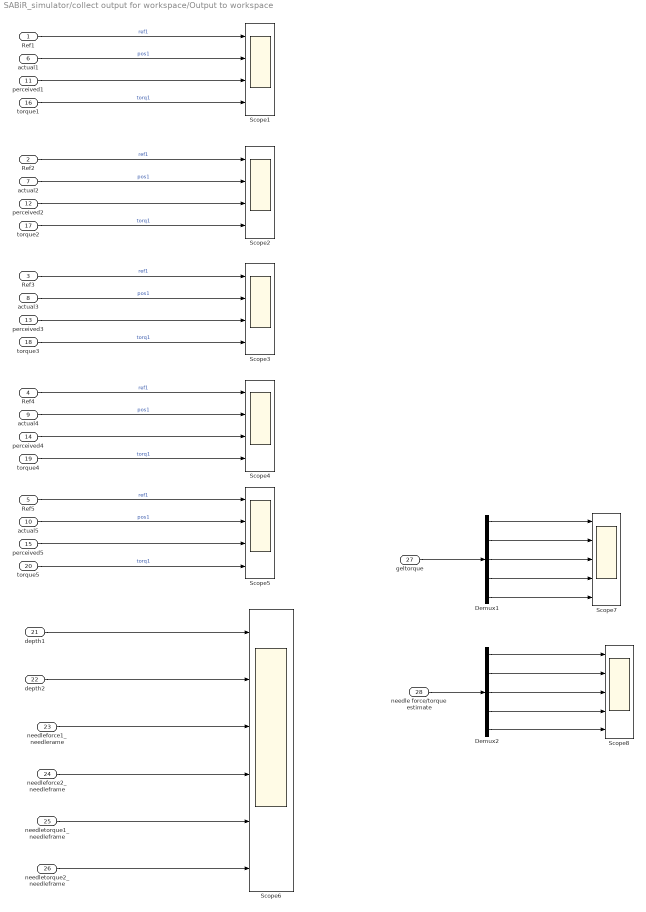
== system SABiR_simulator/collect output for workspace/Output to workspace  ==
  Ref1 : Inport
  Ref2 : Inport  Port=2
  Ref3 : Inport  Port=3
  Ref4 : Inport  Port=4
  Ref5 : Inport  Port=5
  actual1 : Inport  Port=6
  actual2 : Inport  Port=7
  actual3 : Inport  Port=8
  actual4 : Inport  Port=9
  actual5 : Inport  Port=10
  perceived1 : Inport  Port=11
  perceived2 : Inport  Port=12
  perceived3 : Inport  Port=13
  perceived4 : Inport  Port=14
  perceived5 : Inport  Port=15
  torque1 : Inport  Port=16
  torque2 : Inport  Port=17
  torque3 : Inport  Port=18
  torque4 : Inport  Port=19
  torque5 : Inport  Port=20
  depth1 : Inport  Port=21
  depth2 : Inport  Port=22
  needleforce1_needlerame : Inport  Port=23
  needleforce2_needleframe : Inport  Port=24
  needletorque1_needleframe : Inport  Port=25
  needletorque2_needleframe : Inport  Port=26
  geltorque : Inport  Port=27
  needle force/torque estimate : Inport  Port=28
  Demux1 : Demux  Outputs=5
  Demux2 : Demux  Outputs=5
  Scope{1..5} (5 alike) : Scope  NumInputPorts=4
      Scope1 settings: TimeRange=31.611  YMin=-0.125~-0.0007~-5~-5  YMax=0.15~0.0007~5~5  SaveName=axis1
      Scope2 settings: TimeRange=31.611  YMin=-0.125~-0.0007~-5~-5  YMax=0.15~0.0007~5~5  SaveName=axis2
      Scope3 settings: TimeRange=31.611  YMin=-0.125~-0.0007~-5~-5  YMax=0.15~0.0007~5~5  SaveName=axis3
      Scope4 settings: TimeRange=31.611  YMin=-0.125~-0.0007~-5~-5  YMax=0.15~0.0007~5~5  SaveName=axis4
      Scope5 settings: TimeRange=31.611  YMin=-0.125~-0.0007~-5~-5  YMax=0.15~0.0007~5~5  SaveName=axis5
  Scope6 : Scope  NumInputPorts=6
      settings: TimeRange=31.611  YMin=-0.125~-0.0007~-5~-5~-5~-5  YMax=0.15~0.0007~5~5~5~5  SaveName=axis6
  Scope7 : Scope  NumInputPorts=5
      settings: TimeRange=31.611  YMin=-0.125~-0.0007~-5~-5~-5  YMax=0.15~0.0007~5~5~5  SaveName=axis7
  Scope8 : Scope  NumInputPorts=5
      settings: TimeRange=31.611  YMin=-0.125~-0.0007~-5~-5~-5  YMax=0.15~0.0007~5~5~5  SaveName=axis8
  wires:
  Ref1/1 -> Scope1/1  "ref1"
  actual1/1 -> Scope1/2  "pos1"
  perceived1/1 -> Scope1/3
  torque1/1 -> Scope1/4  "torq1"
  Ref2/1 -> Scope2/1  "ref1"
  actual2/1 -> Scope2/2  "pos1"
  perceived2/1 -> Scope2/3
  torque2/1 -> Scope2/4  "torq1"
  Ref3/1 -> Scope3/1  "ref1"
  actual3/1 -> Scope3/2  "pos1"
  perceived3/1 -> Scope3/3
  torque3/1 -> Scope3/4  "torq1"
  Ref4/1 -> Scope4/1  "ref1"
  actual4/1 -> Scope4/2  "pos1"
  perceived4/1 -> Scope4/3
  torque4/1 -> Scope4/4  "torq1"
  Ref5/1 -> Scope5/1  "ref1"
  actual5/1 -> Scope5/2  "pos1"
  perceived5/1 -> Scope5/3
  torque5/1 -> Scope5/4  "torq1"
  depth1/1 -> Scope6/1
  depth2/1 -> Scope6/2
  needleforce1_needlerame/1 -> Scope6/3
  needleforce2_needleframe/1 -> Scope6/4
  needletorque1_needleframe/1 -> Scope6/5
  needletorque2_needleframe/1 -> Scope6/6
  Demux1/1 -> Scope7/1
  Demux1/2 -> Scope7/2
  Demux1/3 -> Scope7/3
  Demux1/4 -> Scope7/4
  Demux1/5 -> Scope7/5
  geltorque/1 -> Demux1/1
  needle force/torque estimate/1 -> Demux2/1
  Demux2/1 -> Scope8/1
  Demux2/2 -> Scope8/2
  Demux2/3 -> Scope8/3
  Demux2/4 -> Scope8/4
  Demux2/5 -> Scope8/5

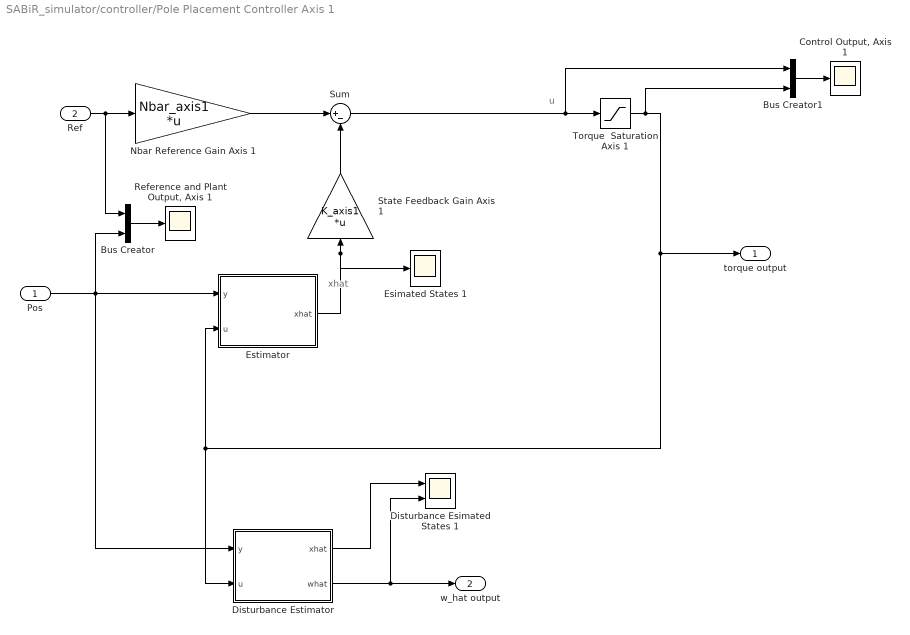
== system SABiR_simulator/controller/Pole Placement Controller Axis 1 ==
  note: u
  note: xhat
  Pos : Inport
  Ref : Inport  Port=2
  Bus Creator : BusCreator  Inputs=2
  Bus Creator1 : BusCreator  Inputs=2
  "Control Output, Axis 1" : Scope
      settings: YMin=-1  YMax=1  SaveName=ScopeData7  MaxDataPoints=500000
  Disturbance Esimated States 1 : Scope  NumInputPorts=2
      settings: YMin=-25~-0.002  YMax=400~0.002  SaveName=ScopeData18  MaxDataPoints=500000
  Disturbance Estimator : Subsystem
  Esimated States 1 : Scope
      settings: YMin=-25  YMax=400  SaveName=ScopeData5  MaxDataPoints=500000
  "Estimator " : Subsystem
  Nbar Reference Gain Axis 1 : Gain  Gain=Nbar_axis1  Multiplication=Matrix(K*u)  SaturateOnIntegerOverflow=on  OutDataTypeStr=Inherit: Same as input  ParamDataTypeStr=Inherit: Same as input
  "Reference and Plant Output, Axis 1" : Scope
      settings: YMin=-0.025  YMax=0.325  MaxDataPoints=500000
  State Feedback Gain Axis 1 : Gain  Gain=K_axis1  Multiplication=Matrix(K*u)  SaturateOnIntegerOverflow=on  OutDataTypeStr=Inherit: Same as input  ParamDataTypeStr=Inherit: Same as input
  Sum : Sum  Inputs=|+-
  Torque  Saturation Axis 1 : Saturate  UpperLimit=SaturationUpperLimit(1)./(1./TorqueConstant(1))  LowerLimit=SaturationLowerLimit(1)./(1./TorqueConstant(1))
  torque output : Outport
  w_hat output : Outport  Port=2
  wires:
  Ref/1 -> Nbar Reference Gain Axis 1/1, Bus Creator/1
  Sum/1 -> Torque  Saturation Axis 1/1, Bus Creator1/1
  Pos/1 -> "Estimator "/1(y), Bus Creator/2, Disturbance Estimator/1(y)
  "Estimator "/1(xhat) -> State Feedback Gain Axis 1/1, Esimated States 1/1
  State Feedback Gain Axis 1/1 -> Sum/2
  Nbar Reference Gain Axis 1/1 -> Sum/1
  Torque  Saturation Axis 1/1 -> torque output/1, "Estimator "/2(u), Disturbance Estimator/2(u), Bus Creator1/2
  Bus Creator/1 -> "Reference and Plant Output, Axis 1"/1
  Bus Creator1/1 -> "Control Output, Axis 1"/1
  Disturbance Estimator/1(xhat) -> Disturbance Esimated States 1/1
  Disturbance Estimator/2(what) -> Disturbance Esimated States 1/2, w_hat output/1

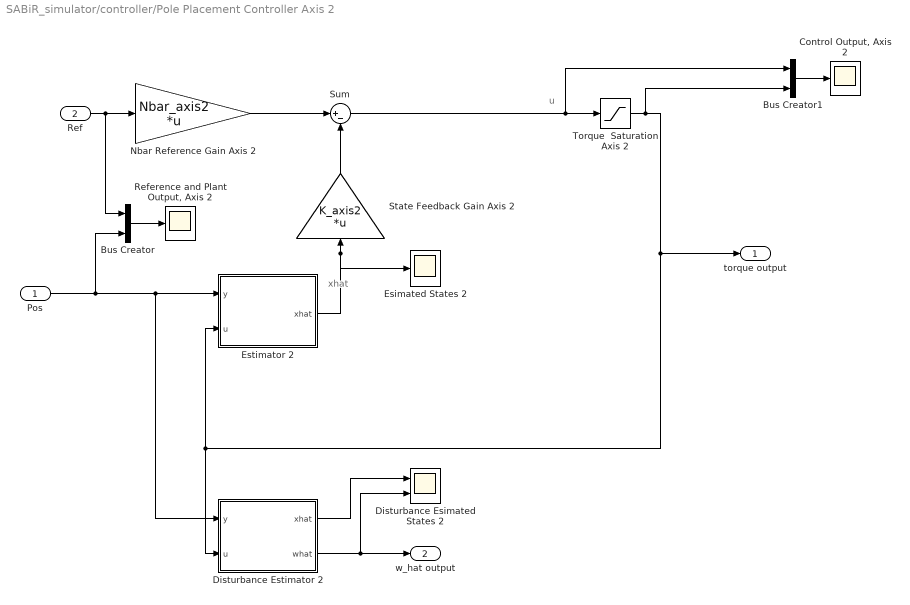
== system SABiR_simulator/controller/Pole Placement Controller Axis 2 ==
  note: u
  note: xhat
  Pos : Inport
  Ref : Inport  Port=2
  Bus Creator : BusCreator  Inputs=2
  Bus Creator1 : BusCreator  Inputs=2
  "Control Output, Axis 2" : Scope
      settings: YMin=-1  YMax=1  SaveName=ScopeData7  MaxDataPoints=500000
  Disturbance Esimated States 2 : Scope  NumInputPorts=2
      settings: YMin=-25~-0.002  YMax=400~0.002  SaveName=ScopeData37  MaxDataPoints=500000
  Disturbance Estimator 2 : Subsystem
  Esimated States 2 : Scope
      settings: YMin=-25  YMax=400  SaveName=ScopeData5  MaxDataPoints=500000
  Estimator 2 : Subsystem
  Nbar Reference Gain Axis 2 : Gain  Gain=Nbar_axis2  Multiplication=Matrix(K*u)  SaturateOnIntegerOverflow=on  OutDataTypeStr=Inherit: Same as input  ParamDataTypeStr=Inherit: Same as input
  "Reference and Plant Output, Axis 2" : Scope
      settings: YMin=-0.025  YMax=0.325  MaxDataPoints=500000
  State Feedback Gain Axis 2 : Gain  Gain=K_axis2  Multiplication=Matrix(K*u)  SaturateOnIntegerOverflow=on  OutDataTypeStr=Inherit: Same as input  ParamDataTypeStr=Inherit: Same as input
  Sum : Sum  Inputs=|+-
  Torque  Saturation Axis 2 : Saturate  UpperLimit=SaturationUpperLimit(2)./(1./TorqueConstant(2))  LowerLimit=SaturationLowerLimit(2)./(1./TorqueConstant(2))
  torque output : Outport
  w_hat output : Outport  Port=2
  wires:
  Ref/1 -> Nbar Reference Gain Axis 2/1, Bus Creator/1
  Sum/1 -> Torque  Saturation Axis 2/1, Bus Creator1/1
  Pos/1 -> Bus Creator/2, Estimator 2/1(y), Disturbance Estimator 2/1(y)
  Estimator 2/1(xhat) -> State Feedback Gain Axis 2/1, Esimated States 2/1
  State Feedback Gain Axis 2/1 -> Sum/2
  Nbar Reference Gain Axis 2/1 -> Sum/1
  Torque  Saturation Axis 2/1 -> torque output/1, Estimator 2/2(u), Disturbance Estimator 2/2(u), Bus Creator1/2
  Bus Creator/1 -> "Reference and Plant Output, Axis 2"/1
  Bus Creator1/1 -> "Control Output, Axis 2"/1
  Disturbance Estimator 2/1(xhat) -> Disturbance Esimated States 2/1
  Disturbance Estimator 2/2(what) -> Disturbance Esimated States 2/2, w_hat output/1

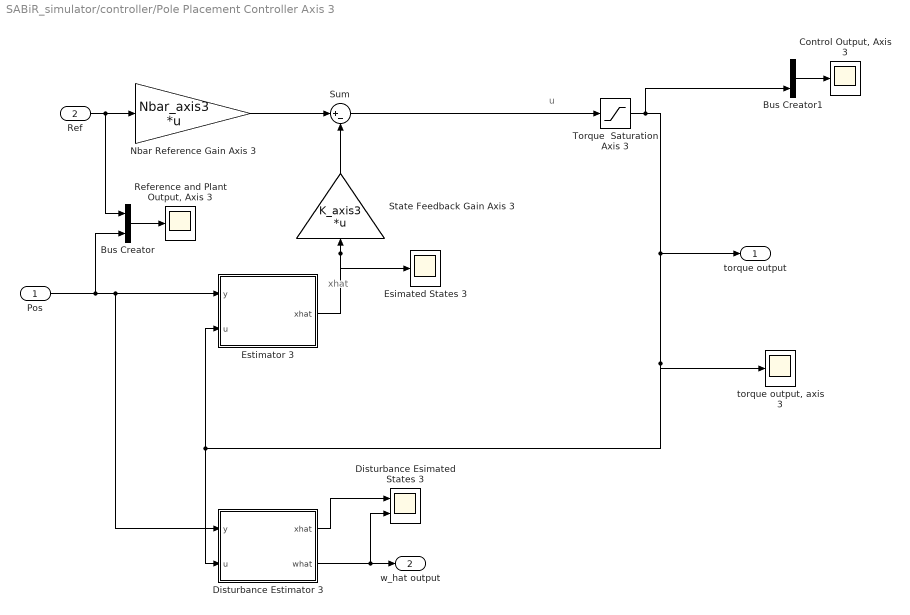
== system SABiR_simulator/controller/Pole Placement Controller Axis 3 ==
  note: u
  note: xhat
  Pos : Inport
  Ref : Inport  Port=2
  Bus Creator : BusCreator  Inputs=2
  Bus Creator1 : BusCreator  Inputs=2
  "Control Output, Axis 3" : Scope
      settings: YMin=-1  YMax=1  SaveName=ScopeData7  MaxDataPoints=500000
  Disturbance Esimated States 3 : Scope  NumInputPorts=2
      settings: YMin=-25~-0.002  YMax=400~0.002  SaveName=ScopeData19  MaxDataPoints=500000
  Disturbance Estimator 3 : Subsystem
  Esimated States 3 : Scope
      settings: YMin=-25  YMax=400  SaveName=ScopeData5  MaxDataPoints=500000
  "Estimator 3 " : Subsystem
  Nbar Reference Gain Axis 3 : Gain  Gain=Nbar_axis3  Multiplication=Matrix(K*u)  SaturateOnIntegerOverflow=on  OutDataTypeStr=Inherit: Same as input  ParamDataTypeStr=Inherit: Same as input
  "Reference and Plant Output, Axis 3" : Scope
      settings: YMin=-0.025  YMax=0.325  MaxDataPoints=500000
  State Feedback Gain Axis 3 : Gain  Gain=K_axis3  Multiplication=Matrix(K*u)  SaturateOnIntegerOverflow=on  OutDataTypeStr=Inherit: Same as input  ParamDataTypeStr=Inherit: Same as input
  Sum : Sum  Inputs=|+-
  Torque  Saturation Axis 3 : Saturate  UpperLimit=SaturationUpperLimit(3)./(1./TorqueConstant(3))  LowerLimit=SaturationLowerLimit(3)./(1./TorqueConstant(3))
  "torque output, axis 3" : Scope
      settings: YMin=-25  YMax=400  SaveName=ScopeData27  MaxDataPoints=500000
  torque output : Outport
  w_hat output : Outport  Port=2
  wires:
  Ref/1 -> Nbar Reference Gain Axis 3/1, Bus Creator/1
  Pos/1 -> Bus Creator/2, "Estimator 3 "/1(y), Disturbance Estimator 3/1(y)
  "Estimator 3 "/1(xhat) -> State Feedback Gain Axis 3/1, Esimated States 3/1
  State Feedback Gain Axis 3/1 -> Sum/2
  Nbar Reference Gain Axis 3/1 -> Sum/1
  Torque  Saturation Axis 3/1 -> torque output/1, "torque output, axis 3"/1, "Estimator 3 "/2(u), Disturbance Estimator 3/2(u), Bus Creator1/2
  Bus Creator/1 -> "Reference and Plant Output, Axis 3"/1
  Bus Creator1/1 -> "Control Output, Axis 3"/1
  Disturbance Estimator 3/2(what) -> w_hat output/1, Disturbance Esimated States 3/2
  Disturbance Estimator 3/1(xhat) -> Disturbance Esimated States 3/1
  Sum/1 -> Torque  Saturation Axis 3/1

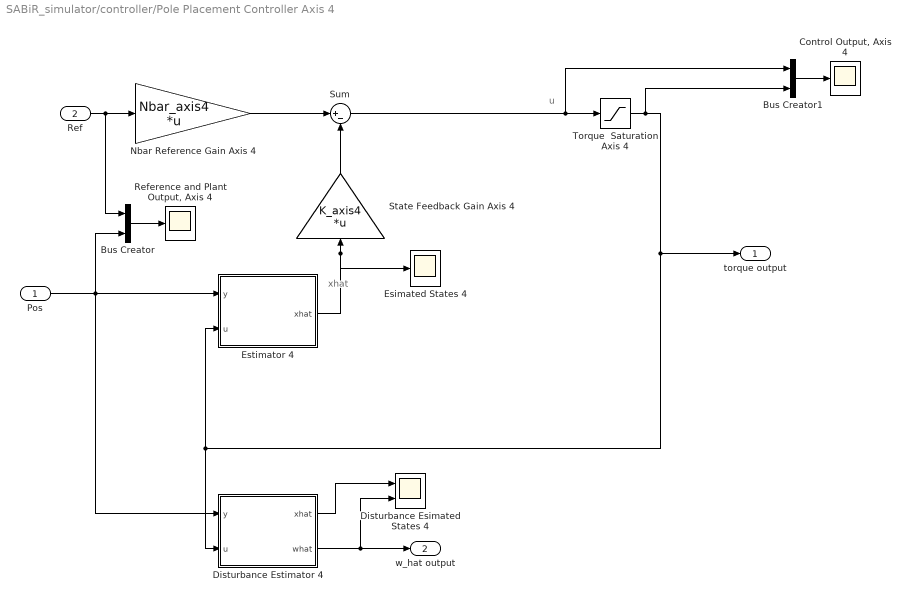
== system SABiR_simulator/controller/Pole Placement Controller Axis 4 ==
  note: u
  note: xhat
  Pos : Inport
  Ref : Inport  Port=2
  Bus Creator : BusCreator  Inputs=2
  Bus Creator1 : BusCreator  Inputs=2
  "Control Output, Axis 4" : Scope
      settings: YMin=-1  YMax=1  SaveName=ScopeData7  MaxDataPoints=500000
  Disturbance Esimated States 4 : Scope  NumInputPorts=2
      settings: YMin=-25~-0.002  YMax=400~0.002  SaveName=ScopeData34  MaxDataPoints=500000
  Disturbance Estimator 4 : Subsystem
  Esimated States 4 : Scope
      settings: YMin=-25  YMax=400  SaveName=ScopeData5  MaxDataPoints=500000
  "Estimator 4 " : Subsystem
  Nbar Reference Gain Axis 4 : Gain  Gain=Nbar_axis4  Multiplication=Matrix(K*u)  SaturateOnIntegerOverflow=on  OutDataTypeStr=Inherit: Same as input  ParamDataTypeStr=Inherit: Same as input
  "Reference and Plant Output, Axis 4" : Scope
      settings: YMin=-0.025  YMax=0.325  MaxDataPoints=500000
  State Feedback Gain Axis 4 : Gain  Gain=K_axis4  Multiplication=Matrix(K*u)  SaturateOnIntegerOverflow=on  OutDataTypeStr=Inherit: Same as input  ParamDataTypeStr=Inherit: Same as input
  Sum : Sum  Inputs=|+-
  Torque  Saturation Axis 4 : Saturate  UpperLimit=SaturationUpperLimit(4)./(1./TorqueConstant(4))  LowerLimit=SaturationLowerLimit(4)./(1./TorqueConstant(4))
  torque output : Outport
  w_hat output : Outport  Port=2
  wires:
  Ref/1 -> Nbar Reference Gain Axis 4/1, Bus Creator/1
  Sum/1 -> Torque  Saturation Axis 4/1, Bus Creator1/1
  Pos/1 -> "Estimator 4 "/1(y), Bus Creator/2, Disturbance Estimator 4/1(y)
  "Estimator 4 "/1(xhat) -> State Feedback Gain Axis 4/1, Esimated States 4/1
  State Feedback Gain Axis 4/1 -> Sum/2
  Nbar Reference Gain Axis 4/1 -> Sum/1
  Torque  Saturation Axis 4/1 -> torque output/1, "Estimator 4 "/2(u), Disturbance Estimator 4/2(u), Bus Creator1/2
  Bus Creator/1 -> "Reference and Plant Output, Axis 4"/1
  Bus Creator1/1 -> "Control Output, Axis 4"/1
  Disturbance Estimator 4/2(what) -> w_hat output/1, Disturbance Esimated States 4/2
  Disturbance Estimator 4/1(xhat) -> Disturbance Esimated States 4/1

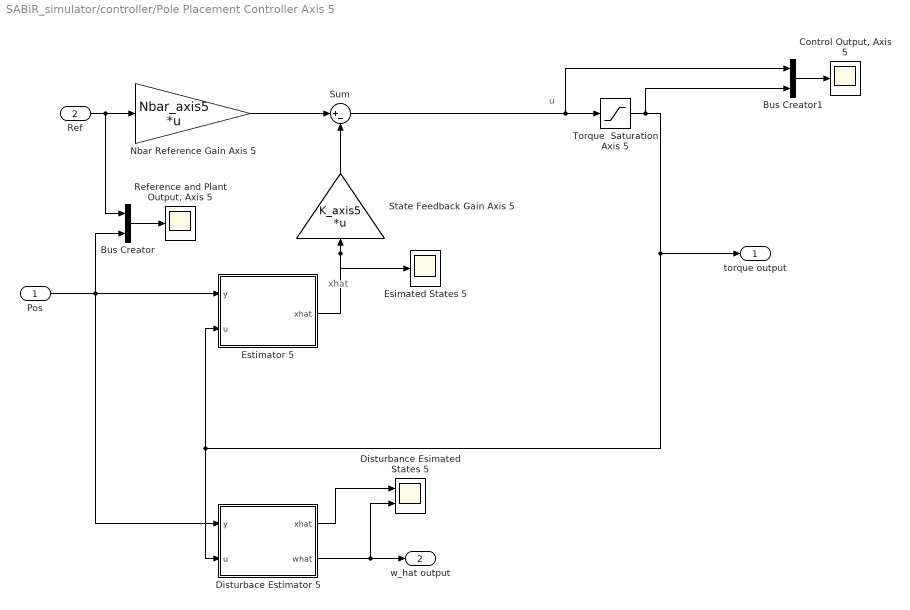
== system SABiR_simulator/controller/Pole Placement Controller Axis 5 ==
  note: u
  note: xhat
  Pos : Inport
  Ref : Inport  Port=2
  Bus Creator : BusCreator  Inputs=2
  Bus Creator1 : BusCreator  Inputs=2
  "Control Output, Axis 5" : Scope
      settings: YMin=-1  YMax=1  SaveName=ScopeData7  MaxDataPoints=500000
  Disturbace Estimator 5 : Subsystem
  Disturbance Esimated States 5 : Scope  NumInputPorts=2
      settings: YMin=-25~-0.002  YMax=400~0.002  SaveName=ScopeData35  MaxDataPoints=500000
  Esimated States 5 : Scope
      settings: YMin=-25  YMax=400  SaveName=ScopeData5  MaxDataPoints=500000
  "Estimator 5 " : Subsystem
  Nbar Reference Gain Axis 5 : Gain  Gain=Nbar_axis5  Multiplication=Matrix(K*u)  SaturateOnIntegerOverflow=on  OutDataTypeStr=Inherit: Same as input  ParamDataTypeStr=Inherit: Same as input
  "Reference and Plant Output, Axis 5" : Scope
      settings: YMin=-0.025  YMax=0.325  MaxDataPoints=500000
  State Feedback Gain Axis 5 : Gain  Gain=K_axis5  Multiplication=Matrix(K*u)  SaturateOnIntegerOverflow=on  OutDataTypeStr=Inherit: Same as input  ParamDataTypeStr=Inherit: Same as input
  Sum : Sum  Inputs=|+-
  Torque  Saturation Axis 5 : Saturate  UpperLimit=SaturationUpperLimit(5)./(1./TorqueConstant(5))  LowerLimit=SaturationLowerLimit(5)./(1./TorqueConstant(5))
  torque output : Outport
  w_hat output : Outport  Port=2
  wires:
  Ref/1 -> Nbar Reference Gain Axis 5/1, Bus Creator/1
  Sum/1 -> Torque  Saturation Axis 5/1, Bus Creator1/1
  Pos/1 -> "Estimator 5 "/1(y), Bus Creator/2, Disturbace Estimator 5/1(y)
  "Estimator 5 "/1(xhat) -> State Feedback Gain Axis 5/1, Esimated States 5/1
  State Feedback Gain Axis 5/1 -> Sum/2
  Nbar Reference Gain Axis 5/1 -> Sum/1
  Torque  Saturation Axis 5/1 -> torque output/1, "Estimator 5 "/2(u), Disturbace Estimator 5/2(u), Bus Creator1/2
  Bus Creator/1 -> "Reference and Plant Output, Axis 5"/1
  Bus Creator1/1 -> "Control Output, Axis 5"/1
  Disturbace Estimator 5/2(what) -> w_hat output/1, Disturbance Esimated States 5/2
  Disturbace Estimator 5/1(xhat) -> Disturbance Esimated States 5/1
